simulink model "hop_simulink"  (R2019b)
settings: Solver=VariableStepAuto  StartTime=0.0  StopTime=10.0  RelTol=1e-3
undefined symbols (not defined in the file or in its folder): sigbuilder_block
libraries: simulink x3, simulink_extras x3, aerolibwind2 x3, shared6dof x1, aerolibatmos2 x1
settings Model: Creator=Lightning  LastModifiedBy=Lightning

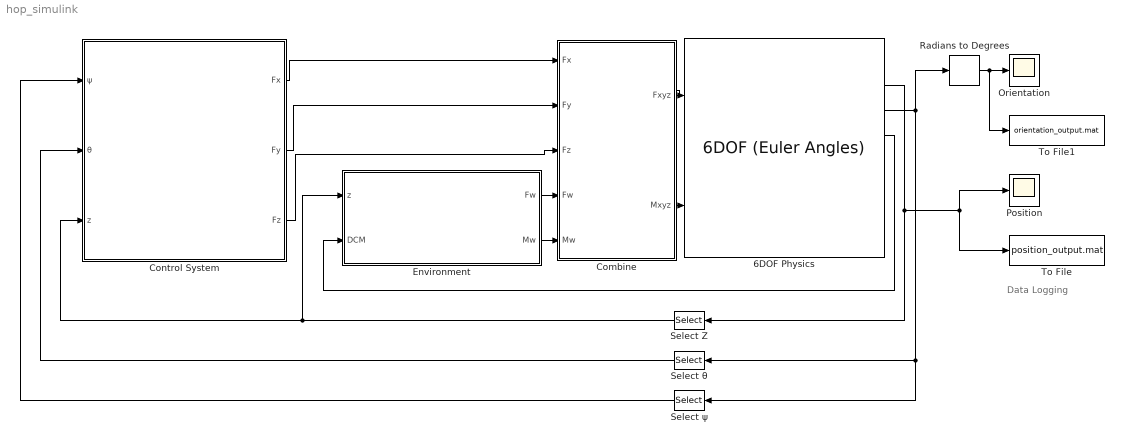
== system hop_simulink ==
  note: Data Logging
  6DOF Physics : shared6dof/6DOF (Euler Angles)  units=Metric (MKS)  mtype=Fixed  rep=Euler Angles  xme_0=[0 0 0]  Vm_0=[0 0 0]  eul_0=[0 0 0]  pm_0=[0 0 0]  mass_0=1.0  mass_e=0.5  mass_f=2.0  inertia=eye(3)  inertia_e=eye(3)  inertia_f=2*eye(3)  k_quat=1.0  vre_flag=on  abi_flag=off  aMode=0  xme_statename=''  Vm_statename=''  eul_statename=''  quat_statename=''  pm_statename=''  mass_statename=''
      settings: SourceProductBaseCode=AE
  Combine : Subsystem
  Control System : Subsystem
  Environment : Subsystem
  Orientation : Scope
  Position : Scope
  Radians to Degrees : simulink_extras/Transformations/Radians to Degrees
  Select Z : Selector  InputPortWidth=3  IndexOptions=Index vector (dialog)  Indices=[3]  OutputSizes=1
  "Select θ " : Selector  InputPortWidth=3  IndexOptions=Index vector (dialog)  Indices=[2]  OutputSizes=1
  Select ψ : Selector  InputPortWidth=3  IndexOptions=Index vector (dialog)  Indices=[1]  OutputSizes=1
  To File : ToFile  Filename=position_output.mat  SaveFormat=Timeseries
  To File1 : ToFile  Filename=orientation_output.mat  SaveFormat=Timeseries
  wires:
  Combine/1(Fxyz) -> 6DOF Physics/1
  Combine/2(Mxyz) -> 6DOF Physics/2
  Control System/1(Fx) -> Combine/1(Fx)
  Control System/2(Fy) -> Combine/2(Fy)
  Control System/3(Fz) -> Combine/3(Fz)
  Select Z/1 -> Control System/3(z), Environment/1(z)
  "Select θ "/1 -> Control System/2(θ)
  Select ψ/1 -> Control System/1(ψ)
  6DOF Physics/3 -> Select ψ/1, "Select θ "/1, Radians to Degrees/1
  Radians to Degrees/1 -> To File1/1, Orientation/1
  6DOF Physics/2 -> Select Z/1, Position/1, To File/1
  Environment/2(Mw) -> Combine/5(Mw)
  Environment/1(Fw) -> Combine/4(Fw)
  6DOF Physics/4 -> Environment/2(DCM)

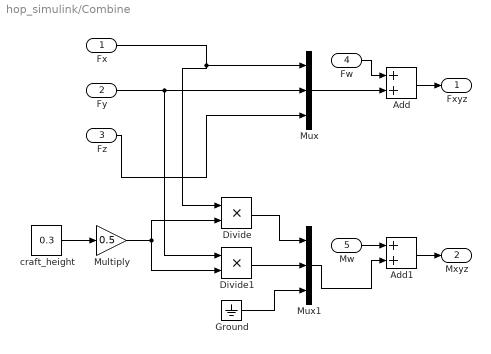
== system hop_simulink/Combine ==
  Fx : Inport
  Fy : Inport  Port=2
  Fz : Inport  Port=3
  Fw : Inport  Port=4
  Mw : Inport  Port=5
  Add : Sum
  Add1 : Sum
  Divide : Product
  Divide1 : Product
  Ground : Ground
  Multiply : Gain  Gain=0.5
  Mux : Mux  Inputs=3
  Mux1 : Mux  Inputs=3
  craft_height : Constant  Value=0.3
  Fxyz : Outport
  Mxyz : Outport  Port=2
  wires:
  Fx/1 -> Divide/1, Mux/1
  Fy/1 -> Divide1/1, Mux/2
  Fz/1 -> Mux/3
  Fw/1 -> Add/1
  Mux/1 -> Add/2
  Add/1 -> Fxyz/1
  Mux1/1 -> Add1/2
  Add1/1 -> Mxyz/1
  Mw/1 -> Add1/1
  Divide/1 -> Mux1/1
  Divide1/1 -> Mux1/2
  Ground/1 -> Mux1/3
  craft_height/1 -> Multiply/1
  Multiply/1 -> Divide1/2, Divide/2

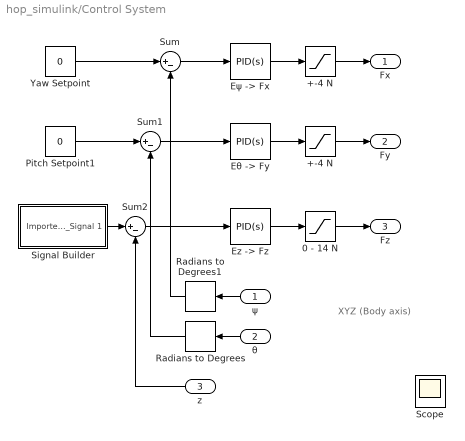
== system hop_simulink/Control System ==
  note: XYZ (Body axis)
  ψ : Inport
  θ : Inport  Port=2
  z : Inport  Port=3
  +-4 N : Saturate  UpperLimit=4  LowerLimit=-4
  "+-4 N " : Saturate  UpperLimit=4  LowerLimit=-4
  0 - 14 N : Saturate  UpperLimit=14  LowerLimit=0
  "Ez -> Fz" : simulink/Continuous/PID Controller  Controller=PID  Form=Parallel  TimeDomain=Continuous-time  SampleTime=-1  IntegratorMethod=Forward Euler  FilterMethod=Forward Euler  ControllerParametersSource=internal  P=21.9594556950671  I=11.7694463428237  D=9.72922647972139  UseFilter=on  N=27.0646894628946  TunerSelectOption=Transfer Function Based (PID Tuner App)  InitialConditionSource=internal  InitialConditionForIntegrator=0  InitialConditionForFilter=0  DifferentiatorICPrevScaledInput=0  ExternalReset=none  TrackingMode=off  Kt=1  LimitOutput=off  UpperSaturationLimit=inf  LowerSaturationLimit=-inf  LinearizeAsGain=on  AntiWindupMode=none  Kb=1  POutMin=[]  POutMax=[]  IOutMin=[]  IOutMax=[]  DOutMin=[]  DOutMax=[]  NOutMin=[]  NOutMax=[]  SumOutMin=[]  SumOutMax=[]  SaturationOutMin=[]  SaturationOutMax=[]  PParamMin=[]  PParamMax=[]  IParamMin=[]  IParamMax=[]  DParamMin=[]  DParamMax=[]  NParamMin=[]  NParamMax=[]  KbParamMin=[]  KbParamMax=[]  KtParamMin=[]  KtParamMax=[]  KbOutMin=[]  KbOutMax=[]  KtOutMin=[]  KtOutMax=[]  IntegratorOutMin=[]  IntegratorOutMax=[]  FilterOutMin=[]  FilterOutMax=[]  SumI1OutMin=[]  SumI1OutMax=[]  SumI2OutMin=[]  SumI2OutMax=[]  SumI3OutMin=[]  SumI3OutMax=[]  SumI4OutMin=[]  SumI4OutMax=[]  SumDOutMin=[]  SumDOutMax=[]  DifferentiatorOutMin=[]  DifferentiatorOutMax=[]  FilterDiffOutCoefMin=[]  FilterDiffOutCoefMax=[]  ReciprocalOutMin=[]  ReciprocalOutMax=[]  SumDenOutMin=[]  SumDenOutMax=[]  SumNumOutMin=[]  SumNumOutMax=[]  DivideOutMin=[]  DivideOutMax=[]  IntegratorContinuousStateAttributes=''  IntegratorStateMustResolveToSignalObject=off  IntegratorRTWStateStorageClass=Auto  FilterContinuousStateAttributes=''  FilterStateMustResolveToSignalObject=off  FilterRTWStateStorageClass=Auto  ParallelPVariant=InternalParameters  IdealPVariant=Disabled  IVariant=InternalParameters  DVariant=InternalParameters  IntegratorVariant=Continuous  SatVariant=Disabled  AWVariant=Passthrough  PCopyVariant=Disabled  TRVariant=Disabled  FdbkBlocksVariant=Forward  IdealPFdbkVariant=Disabled  SatFdbkVariant=Disabled  DerivativeFilterVariant=ContFilter  NVariant=InternalParameters  NCopyVariant=Disabled  FilterICVariant=InternalICsFilter  IntegratorICVariant=InternalICs  ExternalResetVariant=Disabled  TRSumVariant=Passthrough  SumFdbkVariant=Disabled  SumVariant=Sum_PID
  "Eθ -> Fy" : simulink/Continuous/PID Controller  Controller=PID  Form=Parallel  TimeDomain=Continuous-time  SampleTime=-1  IntegratorMethod=Forward Euler  FilterMethod=Forward Euler  ControllerParametersSource=internal  P=10.3851067196303  I=1.4577525381907  D=2.01781775273091  UseFilter=on  N=16.5093040881366  TunerSelectOption=Transfer Function Based (PID Tuner App)  InitialConditionSource=internal  InitialConditionForIntegrator=0  InitialConditionForFilter=0  DifferentiatorICPrevScaledInput=0  ExternalReset=none  TrackingMode=off  Kt=1  LimitOutput=off  UpperSaturationLimit=inf  LowerSaturationLimit=-inf  LinearizeAsGain=on  AntiWindupMode=none  Kb=1  POutMin=[]  POutMax=[]  IOutMin=[]  IOutMax=[]  DOutMin=[]  DOutMax=[]  NOutMin=[]  NOutMax=[]  SumOutMin=[]  SumOutMax=[]  SaturationOutMin=[]  SaturationOutMax=[]  PParamMin=[]  PParamMax=[]  IParamMin=[]  IParamMax=[]  DParamMin=[]  DParamMax=[]  NParamMin=[]  NParamMax=[]  KbParamMin=[]  KbParamMax=[]  KtParamMin=[]  KtParamMax=[]  KbOutMin=[]  KbOutMax=[]  KtOutMin=[]  KtOutMax=[]  IntegratorOutMin=[]  IntegratorOutMax=[]  FilterOutMin=[]  FilterOutMax=[]  SumI1OutMin=[]  SumI1OutMax=[]  SumI2OutMin=[]  SumI2OutMax=[]  SumI3OutMin=[]  SumI3OutMax=[]  SumI4OutMin=[]  SumI4OutMax=[]  SumDOutMin=[]  SumDOutMax=[]  DifferentiatorOutMin=[]  DifferentiatorOutMax=[]  FilterDiffOutCoefMin=[]  FilterDiffOutCoefMax=[]  ReciprocalOutMin=[]  ReciprocalOutMax=[]  SumDenOutMin=[]  SumDenOutMax=[]  SumNumOutMin=[]  SumNumOutMax=[]  DivideOutMin=[]  DivideOutMax=[]  IntegratorContinuousStateAttributes=''  IntegratorStateMustResolveToSignalObject=off  IntegratorRTWStateStorageClass=Auto  FilterContinuousStateAttributes=''  FilterStateMustResolveToSignalObject=off  FilterRTWStateStorageClass=Auto  ParallelPVariant=InternalParameters  IdealPVariant=Disabled  IVariant=InternalParameters  DVariant=InternalParameters  IntegratorVariant=Continuous  SatVariant=Disabled  AWVariant=Passthrough  PCopyVariant=Disabled  TRVariant=Disabled  FdbkBlocksVariant=Forward  IdealPFdbkVariant=Disabled  SatFdbkVariant=Disabled  DerivativeFilterVariant=ContFilter  NVariant=InternalParameters  NCopyVariant=Disabled  FilterICVariant=InternalICsFilter  IntegratorICVariant=InternalICs  ExternalResetVariant=Disabled  TRSumVariant=Passthrough  SumFdbkVariant=Disabled  SumVariant=Sum_PID
  "Eψ -> Fx" : simulink/Continuous/PID Controller  Controller=PID  Form=Parallel  TimeDomain=Continuous-time  SampleTime=-1  IntegratorMethod=Forward Euler  FilterMethod=Forward Euler  ControllerParametersSource=internal  P=10.3851067196303  I=1.4577525381907  D=2.01781775273091  UseFilter=on  N=16.5093040881366  TunerSelectOption=Transfer Function Based (PID Tuner App)  InitialConditionSource=internal  InitialConditionForIntegrator=0  InitialConditionForFilter=0  DifferentiatorICPrevScaledInput=0  ExternalReset=none  TrackingMode=off  Kt=1  LimitOutput=off  UpperSaturationLimit=inf  LowerSaturationLimit=-inf  LinearizeAsGain=on  AntiWindupMode=none  Kb=1  POutMin=[]  POutMax=[]  IOutMin=[]  IOutMax=[]  DOutMin=[]  DOutMax=[]  NOutMin=[]  NOutMax=[]  SumOutMin=[]  SumOutMax=[]  SaturationOutMin=[]  SaturationOutMax=[]  PParamMin=[]  PParamMax=[]  IParamMin=[]  IParamMax=[]  DParamMin=[]  DParamMax=[]  NParamMin=[]  NParamMax=[]  KbParamMin=[]  KbParamMax=[]  KtParamMin=[]  KtParamMax=[]  KbOutMin=[]  KbOutMax=[]  KtOutMin=[]  KtOutMax=[]  IntegratorOutMin=[]  IntegratorOutMax=[]  FilterOutMin=[]  FilterOutMax=[]  SumI1OutMin=[]  SumI1OutMax=[]  SumI2OutMin=[]  SumI2OutMax=[]  SumI3OutMin=[]  SumI3OutMax=[]  SumI4OutMin=[]  SumI4OutMax=[]  SumDOutMin=[]  SumDOutMax=[]  DifferentiatorOutMin=[]  DifferentiatorOutMax=[]  FilterDiffOutCoefMin=[]  FilterDiffOutCoefMax=[]  ReciprocalOutMin=[]  ReciprocalOutMax=[]  SumDenOutMin=[]  SumDenOutMax=[]  SumNumOutMin=[]  SumNumOutMax=[]  DivideOutMin=[]  DivideOutMax=[]  IntegratorContinuousStateAttributes=''  IntegratorStateMustResolveToSignalObject=off  IntegratorRTWStateStorageClass=Auto  FilterContinuousStateAttributes=''  FilterStateMustResolveToSignalObject=off  FilterRTWStateStorageClass=Auto  ParallelPVariant=InternalParameters  IdealPVariant=Disabled  IVariant=InternalParameters  DVariant=InternalParameters  IntegratorVariant=Continuous  SatVariant=Disabled  AWVariant=Passthrough  PCopyVariant=Disabled  TRVariant=Disabled  FdbkBlocksVariant=Forward  IdealPFdbkVariant=Disabled  SatFdbkVariant=Disabled  DerivativeFilterVariant=ContFilter  NVariant=InternalParameters  NCopyVariant=Disabled  FilterICVariant=InternalICsFilter  IntegratorICVariant=InternalICs  ExternalResetVariant=Disabled  TRSumVariant=Passthrough  SumFdbkVariant=Disabled  SumVariant=Sum_PID
  Pitch Setpoint1 : Constant  Value=0
  Radians to Degrees : simulink_extras/Transformations/Radians to Degrees
  Radians to Degrees1 : simulink_extras/Transformations/Radians to Degrees
  Scope : Scope
  Signal Builder : Subsystem  Tag=STV Subsys  LoadFcn=sigbuilder_block('load');  StartFcn=sigbuilder_block('start');  StopFcn=sigbuilder_block('stop');  ClipboardFcn=sigbuilder_block('clipboard');  mask(Sigbuilder block){tuvar=[0:10]}
      mask help: Simulink:masks:SigbuilderBlock_MD
      mask init:
      | if ~strcmp(get_param(bdroot(gcbh),'SimulationStatus'),'stopped') tuvar = sigbuilder_block('maskInit'); end
      settings: CopyFcn=sigbuilder_block('copy');  DeleteFcn=sigbuilder_block('delete');  ModelCloseFcn=sigbuilder_block('modelClose');  PreSaveFcn=sigbuilder_block('preSave');  PauseFcn=sigbuilder_block('pause');  ContinueFcn=sigbuilder_block('continue');  NameChangeFcn=sigbuilder_block('namechange');  OpenFcn=sigbuilder_block('open',[437.6 199.2 550.4 400 ]);  CloseFcn=sigbuilder_block('close');
      mask Display: plot(0, 0, 100, 100,[2, 2, 32, 32, 2], [68, 8, 8, 68, 68],[32, 2], [38, 38], [32, 19, 2],[53, 60, 44], [32, 17, 17, 2],[16, 16, 31, 31]);txt = getActiveGroup(gcbh);text(2, 100, txt,'verticalAlignment', 'top');
  Sum : Sum  Inputs=|+-
  Sum1 : Sum  Inputs=|+-
  Sum2 : Sum  Inputs=|+-
  Yaw Setpoint : Constant  Value=0
  Fx : Outport
  Fy : Outport  Port=2
  Fz : Outport  Port=3
  wires:
  Pitch Setpoint1/1 -> Sum1/1
  Sum1/1 -> "Eθ -> Fy"/1
  z/1 -> Sum2/2
  Signal Builder/1(Imported_Signal 1) -> Sum2/1
  Radians to Degrees1/1 -> Sum/2
  Sum/1 -> "Eψ -> Fx"/1
  Yaw Setpoint/1 -> Sum/1
  Radians to Degrees/1 -> Sum1/2
  Sum2/1 -> "Ez -> Fz"/1
  "Ez -> Fz"/1 -> 0 - 14 N/1
  "Eθ -> Fy"/1 -> +-4 N/1
  "Eψ -> Fx"/1 -> "+-4 N "/1
  0 - 14 N/1 -> Fz/1
  +-4 N/1 -> Fy/1
  "+-4 N "/1 -> Fx/1
  θ/1 -> Radians to Degrees/1
  ψ/1 -> Radians to Degrees1/1

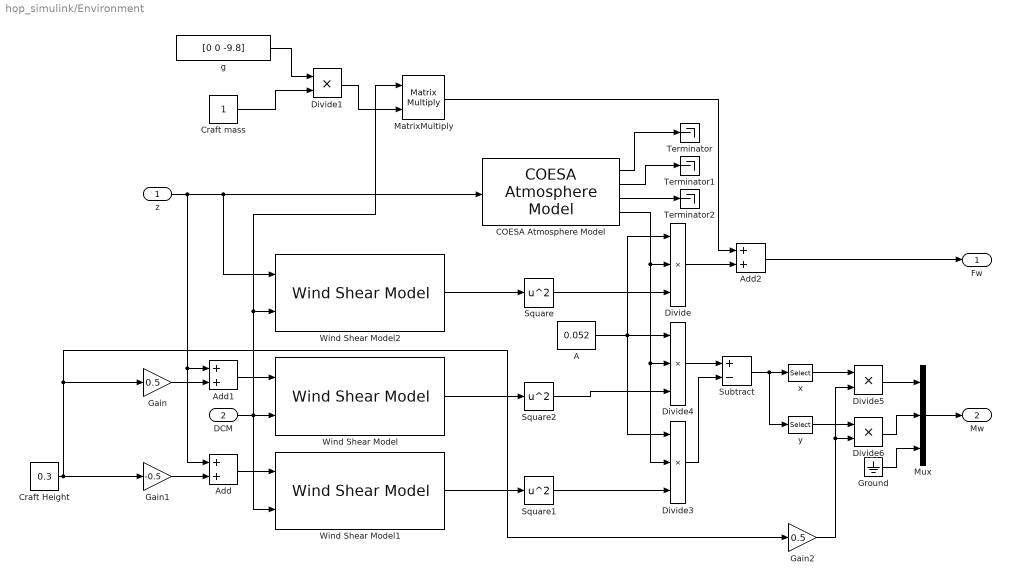
== system hop_simulink/Environment ==
  z : Inport
  DCM : Inport  Port=2
  A : Constant  Value=0.052
  Add : Sum
  Add1 : Sum
  Add2 : Sum
  COESA Atmosphere Model : aerolibatmos2/COESA Atmosphere Model  units=Metric (MKS)  spec=1976 COESA-extended U.S. Standard Atmosphere  model=Profile  profile_var=High temperature  profile_percent=1%  profile_alt=5 km (16404 ft)  envelope_var=High temperature  envelope_percent=1%  action=Warning
  Craft Height : Constant  Value=0.3
  Craft mass : Constant
  Divide : Product  Inputs=3
  Divide1 : Product  Inputs=**
  Divide3 : Product  Inputs=3
  Divide4 : Product  Inputs=3
  Divide5 : Product
  Divide6 : Product
  Gain : Gain  Gain=0.5
  Gain1 : Gain  Gain=-0.5
  Gain2 : Gain  Gain=0.5
  Ground : Ground
  MatrixMultiply : Product  Multiplication=Matrix(*)
  Mux : Mux  Inputs=3
  Square : Math  Operator=square  SignedPower=off  SaturateOnIntegerOverflow=on
  Square1 : Math  Operator=square  SignedPower=off  SaturateOnIntegerOverflow=on
  Square2 : Math  Operator=square  SignedPower=off  SaturateOnIntegerOverflow=on
  Subtract : Sum  Inputs=+-
  Terminator : Terminator
  Terminator1 : Terminator
  Terminator2 : Terminator
  Wind Shear Model : aerolibwind2/Wind Shear Model  units=Metric (MKS)  phase=Category C - Terminal Flight Phase  W_20=3  Wdeg=30
      settings: SourceProductName=Aerospace Blockset
  Wind Shear Model1 : aerolibwind2/Wind Shear Model  units=Metric (MKS)  phase=Category C - Terminal Flight Phase  W_20=3  Wdeg=30
      settings: SourceProductName=Aerospace Blockset
  Wind Shear Model2 : aerolibwind2/Wind Shear Model  units=Metric (MKS)  phase=Category C - Terminal Flight Phase  W_20=3  Wdeg=30
      settings: SourceProductName=Aerospace Blockset
  g : Constant  Value=[0 0 -9.8]
  x : Selector  InputPortWidth=3  IndexOptions=Index vector (dialog)  Indices=[1]  OutputSizes=1
  y : Selector  InputPortWidth=3  IndexOptions=Index vector (dialog)  Indices=[2]  OutputSizes=1
  Fw : Outport
  Mw : Outport  Port=2
  wires:
  z/1 -> Wind Shear Model2/1, COESA Atmosphere Model/1, Add1/1, Add/1
  Mux/1 -> Mw/1
  Divide6/1 -> Mux/2
  Divide3/1 -> Subtract/2
  COESA Atmosphere Model/4 -> Divide4/2, Divide3/2, Divide/2
  Ground/1 -> Mux/3
  x/1 -> Divide5/1
  Divide5/1 -> Mux/1
  Wind Shear Model/1 -> Square2/1
  y/1 -> Divide6/1
  Divide4/1 -> Subtract/1
  Square2/1 -> Divide4/3
  Wind Shear Model1/1 -> Square1/1
  Craft Height/1 -> Gain/1, Gain2/1, Gain1/1
  Square1/1 -> Divide3/3
  Add/1 -> Wind Shear Model1/1
  Gain1/1 -> Add/2
  Gain/1 -> Add1/2
  Add1/1 -> Wind Shear Model/1
  Square/1 -> Divide/3
  Wind Shear Model2/1 -> Square/1
  COESA Atmosphere Model/3 -> Terminator2/1
  COESA Atmosphere Model/2 -> Terminator1/1
  COESA Atmosphere Model/1 -> Terminator/1
  Divide/1 -> Add2/2
  Gain2/1 -> Divide5/2, Divide6/2
  Subtract/1 -> x/1, y/1
  A/1 -> Divide3/1, Divide4/1, Divide/1
  g/1 -> Divide1/1
  Craft mass/1 -> Divide1/2
  Divide1/1 -> MatrixMultiply/2
  DCM/1 -> Wind Shear Model1/2, MatrixMultiply/1, Wind Shear Model2/2, Wind Shear Model/2
  MatrixMultiply/1 -> Add2/1
  Add2/1 -> Fw/1

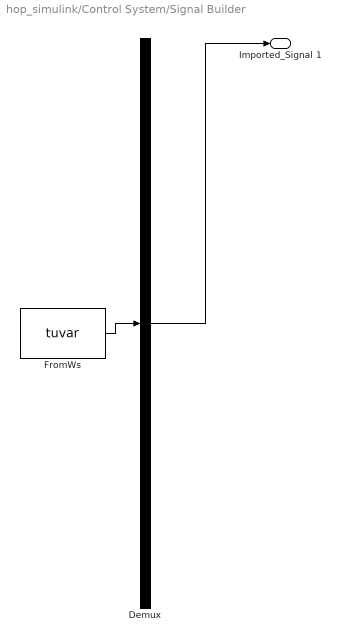
== system hop_simulink/Control System/Signal Builder ==
  Demux : Demux  Tag=STV Demux  Outputs=1
  FromWs : FromWorkspace  Tag=STV FromWs  VariableName=tuvar  SampleTime=0
      SigBuilderData=|
      | common.afterFinalStr = 'Extrapolate'
      | common.sampleTime = 0
      | dataSet.timeRange = [0 10]
      | dataSet.name = 'Imported_Group 1'
      | sbobj.Groups.Name = 'Imported_Group 1'
      | sbobj.Groups.Signals.Name = 'Imported_Signal 1'
      | sbobj.Groups.Signals.XData = [0 2 4 6 8 10]
      | sbobj.Groups.Signals.YData = [0 5 5 3 0.1 0.002]
  Imported_Signal 1 : Outport  Tag=STV Outport
  wires:
  Demux/1 -> Imported_Signal 1/1
  FromWs/1 -> Demux/1
